simulink model "pendulum"  (R2016b)
settings: Solver=VariableStepAuto  StartTime=0.0  StopTime=10.0  RelTol=1e-3
values from neighbouring files (symbols this model uses):
  Bp = 0.03    [Pendulumm.m]
  g = 9.81    [Pendulumm.m]
  L = 0.8    [Pendulumm.m]
  m = 0.3    [Pendulumm.m]
settings Model: Creator=leekunhwee  LastModifiedBy=Alex

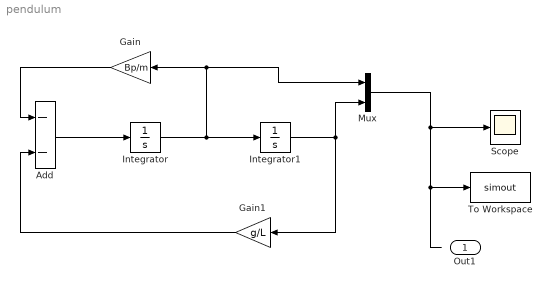
== system pendulum ==
  Add : Sum  Inputs=--
  Gain : Gain  Gain=Bp/m
  Gain1 : Gain  Gain=g/L
  Integrator : Integrator
  Integrator1 : Integrator  InitialCondition=1
  Mux : Mux  Inputs=2
  Scope : Scope
  To Workspace : ToWorkspace  VariableName=simout  SampleTime=-1
  Out1 : Outport
  wires:
  Add/1 -> Integrator/1
  Integrator/1 -> Mux/1, Gain/1, Integrator1/1
  Gain/1 -> Add/1
  Gain1/1 -> Add/2
  Integrator1/1 -> Mux/2, Gain1/1
  Mux/1 -> To Workspace/1, Scope/1
